simulink model "Battery_50kw_AC_500KW_400V_pruebas_2020_2_individual"  (R2020b)
settings: Solver=VariableStepAuto  StartTime=0.0  StopTime=0.4  RelTol=1e-3
InitFcn:
  | Ts=100e-6;
  | Timer=0.001;
StartFcn:
  | Ts=100e-6;
  | Timer=0.001;
undefined symbols (not defined in the file or in its folder): Ion, Lithium
libraries: powerlib x44, powerlib_meascontrol x16, slpidlib x10, simulink x5, electricdrivelib x1
(part 2 of 2)

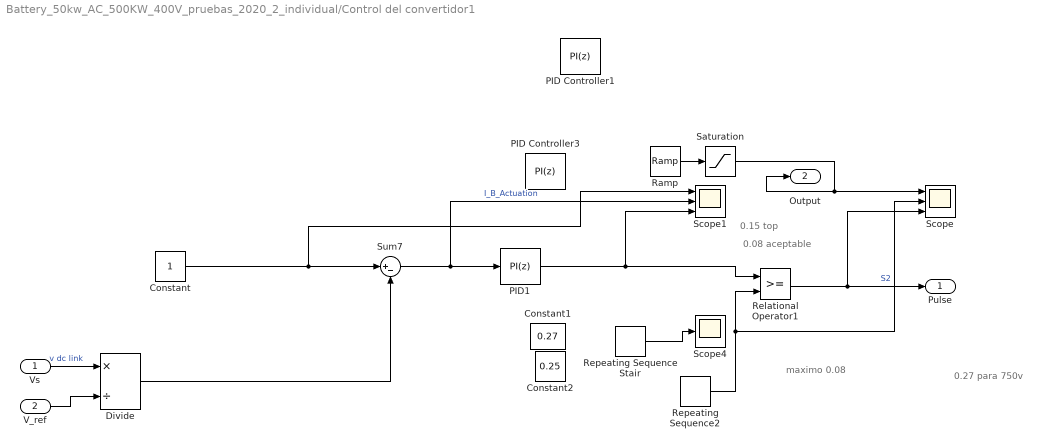
== system Battery_50kw_AC_500KW_400V_pruebas_2020_2_individual/Control del convertidor1 ==
  note: 0.08 aceptable
  note: 0.15 top
  note: 0.27 para 750v
  note: maximo 0.08
  Vs : Inport
  V_ref : Inport  Port=2
  Constant : Constant
  Constant1 : Constant  Value=0.27
  Constant2 : Constant  Value=0.25
  Divide : Product  Inputs=*/
  PID Controller1 : slpidlib/PID Controller  Controller=PI  Form=Parallel  TimeDomain=Discrete-time  UseExternalTs=off  SampleTime=Ts  IntegratorMethod=Forward Euler  FilterMethod=Forward Euler  ControllerParametersSource=internal  P=0.01  I=0.02  D=0  UseFilter=on  N=100  TunerSelectOption=Transfer Function Based (PID Tuner App)  InitialConditionSource=internal  InitialConditionForIntegrator=0  InitialConditionForFilter=0  DifferentiatorICPrevScaledInput=0  ExternalReset=none  TrackingMode=off  Kt=1  LimitOutput=on  SatLimitsSource=internal  UpperSaturationLimit=0.95  LowerSaturationLimit=0  LinearizeAsGain=on  AntiWindupMode=clamping  Kb=1  POutMin=[]  POutMax=[]  IOutMin=[]  IOutMax=[]  DOutMin=[]  DOutMax=[]  NOutMin=[]  NOutMax=[]  SumOutMin=[]  SumOutMax=[]  SaturationOutMin=[]  SaturationOutMax=[]  PParamMin=[]  PParamMax=[]  IParamMin=[]  IParamMax=[]  DParamMin=[]  DParamMax=[]  NParamMin=[]  NParamMax=[]  KbParamMin=[]  KbParamMax=[]  KtParamMin=[]  KtParamMax=[]  KbOutMin=[]  KbOutMax=[]  KtOutMin=[]  KtOutMax=[]  IntegratorOutMin=[]  IntegratorOutMax=[]  FilterOutMin=[]  FilterOutMax=[]  SumI1OutMin=[]  SumI1OutMax=[]  SumI2OutMin=[]  SumI2OutMax=[]  SumI3OutMin=[]  SumI3OutMax=[]  SumI4OutMin=[]  SumI4OutMax=[]  SumDOutMin=[]  SumDOutMax=[]  DifferentiatorOutMin=[]  DifferentiatorOutMax=[]  FilterDiffOutCoefMin=[]  FilterDiffOutCoefMax=[]  ReciprocalOutMin=[]  ReciprocalOutMax=[]  SumDenOutMin=[]  SumDenOutMax=[]  SumNumOutMin=[]  SumNumOutMax=[]  DivideOutMin=[]  DivideOutMax=[]  UdiffTsProdOutMin=[]  UdiffTsProdOutMax=[]  NTsProdOutMin=[]  NTsProdOutMax=[]  UintegralTsProdOutMin=[]  UintegralTsProdOutMax=[]  UngainTsProdOutMin=[]  UngainTsProdOutMax=[]  IntegratorContinuousStateAttributes=''  IntegratorStateMustResolveToSignalObject=off  IntegratorRTWStateStorageClass=Auto  FilterContinuousStateAttributes=''  FilterStateMustResolveToSignalObject=off  FilterRTWStateStorageClass=Auto  ParallelPVariant=InternalParameters  IdealPVariant=Disabled  IVariant=InternalParameters  DVariant=Disabled  IntegratorVariant=Discrete  SatVariant=Enabled  AWVariant=DiscClampingParallel  PCopyVariant=Disabled  TRVariant=Disabled  FdbkBlocksVariant=Forward  IdealPFdbkVariant=Disabled  SatFdbkVariant=Disabled  DerivativeFilterVariant=Disabled  NVariant=Disabled  NCopyVariant=Disabled_SignalSpec  FilterICVariant=Disabled  IntegratorICVariant=InternalICs  ExternalResetVariant=Disabled  TRSumVariant=Passthrough  SumFdbkVariant=Disabled  SumVariant=Sum_PI  TsampFilterVariant=InternalTs  TsampNgainVariant=Passthrough  TsampIntegralVariant=Passthrough  ExternalSaturationOutDataTypeStr=Inherit: Same as second input
  PID Controller3 : slpidlib/PID Controller  Controller=PI  Form=Parallel  TimeDomain=Discrete-time  UseExternalTs=off  SampleTime=Ts  IntegratorMethod=Forward Euler  FilterMethod=Forward Euler  ControllerParametersSource=internal  P=0.001  I=0.02  D=0  UseFilter=on  N=100  TunerSelectOption=Transfer Function Based (PID Tuner App)  InitialConditionSource=internal  InitialConditionForIntegrator=0  InitialConditionForFilter=0  DifferentiatorICPrevScaledInput=0  ExternalReset=none  TrackingMode=off  Kt=1  LimitOutput=on  SatLimitsSource=internal  UpperSaturationLimit=0.95  LowerSaturationLimit=0  LinearizeAsGain=on  AntiWindupMode=clamping  Kb=1  POutMin=[]  POutMax=[]  IOutMin=[]  IOutMax=[]  DOutMin=[]  DOutMax=[]  NOutMin=[]  NOutMax=[]  SumOutMin=[]  SumOutMax=[]  SaturationOutMin=[]  SaturationOutMax=[]  PParamMin=[]  PParamMax=[]  IParamMin=[]  IParamMax=[]  DParamMin=[]  DParamMax=[]  NParamMin=[]  NParamMax=[]  KbParamMin=[]  KbParamMax=[]  KtParamMin=[]  KtParamMax=[]  KbOutMin=[]  KbOutMax=[]  KtOutMin=[]  KtOutMax=[]  IntegratorOutMin=[]  IntegratorOutMax=[]  FilterOutMin=[]  FilterOutMax=[]  SumI1OutMin=[]  SumI1OutMax=[]  SumI2OutMin=[]  SumI2OutMax=[]  SumI3OutMin=[]  SumI3OutMax=[]  SumI4OutMin=[]  SumI4OutMax=[]  SumDOutMin=[]  SumDOutMax=[]  DifferentiatorOutMin=[]  DifferentiatorOutMax=[]  FilterDiffOutCoefMin=[]  FilterDiffOutCoefMax=[]  ReciprocalOutMin=[]  ReciprocalOutMax=[]  SumDenOutMin=[]  SumDenOutMax=[]  SumNumOutMin=[]  SumNumOutMax=[]  DivideOutMin=[]  DivideOutMax=[]  UdiffTsProdOutMin=[]  UdiffTsProdOutMax=[]  NTsProdOutMin=[]  NTsProdOutMax=[]  UintegralTsProdOutMin=[]  UintegralTsProdOutMax=[]  UngainTsProdOutMin=[]  UngainTsProdOutMax=[]  IntegratorContinuousStateAttributes=''  IntegratorStateMustResolveToSignalObject=off  IntegratorRTWStateStorageClass=Auto  FilterContinuousStateAttributes=''  FilterStateMustResolveToSignalObject=off  FilterRTWStateStorageClass=Auto  ParallelPVariant=InternalParameters  IdealPVariant=Disabled  IVariant=InternalParameters  DVariant=Disabled  IntegratorVariant=Discrete  SatVariant=Enabled  AWVariant=DiscClampingParallel  PCopyVariant=Disabled  TRVariant=Disabled  FdbkBlocksVariant=Forward  IdealPFdbkVariant=Disabled  SatFdbkVariant=Disabled  DerivativeFilterVariant=Disabled  NVariant=Disabled  NCopyVariant=Disabled_SignalSpec  FilterICVariant=Disabled  IntegratorICVariant=InternalICs  ExternalResetVariant=Disabled  TRSumVariant=Passthrough  SumFdbkVariant=Disabled  SumVariant=Sum_PI  TsampFilterVariant=InternalTs  TsampNgainVariant=Passthrough  TsampIntegralVariant=Passthrough  ExternalSaturationOutDataTypeStr=Inherit: Same as second input
  PID1 : slpidlib/PID Controller  Controller=PI  Form=Parallel  TimeDomain=Discrete-time  UseExternalTs=off  SampleTime=Ts  IntegratorMethod=Forward Euler  FilterMethod=Forward Euler  ControllerParametersSource=internal  P=0.7  I=5  D=0  UseFilter=on  N=100  TunerSelectOption=Transfer Function Based (PID Tuner App)  InitialConditionSource=internal  InitialConditionForIntegrator=0.26  InitialConditionForFilter=0  DifferentiatorICPrevScaledInput=0  ExternalReset=none  TrackingMode=off  Kt=1  LimitOutput=on  SatLimitsSource=internal  UpperSaturationLimit=0.97  LowerSaturationLimit=0  LinearizeAsGain=on  AntiWindupMode=clamping  Kb=1  POutMin=[]  POutMax=[]  IOutMin=[]  IOutMax=[]  DOutMin=[]  DOutMax=[]  NOutMin=[]  NOutMax=[]  SumOutMin=[]  SumOutMax=[]  SaturationOutMin=[]  SaturationOutMax=[]  PParamMin=[]  PParamMax=[]  IParamMin=[]  IParamMax=[]  DParamMin=[]  DParamMax=[]  NParamMin=[]  NParamMax=[]  KbParamMin=[]  KbParamMax=[]  KtParamMin=[]  KtParamMax=[]  KbOutMin=[]  KbOutMax=[]  KtOutMin=[]  KtOutMax=[]  IntegratorOutMin=[]  IntegratorOutMax=[]  FilterOutMin=[]  FilterOutMax=[]  SumI1OutMin=[]  SumI1OutMax=[]  SumI2OutMin=[]  SumI2OutMax=[]  SumI3OutMin=[]  SumI3OutMax=[]  SumI4OutMin=[]  SumI4OutMax=[]  SumDOutMin=[]  SumDOutMax=[]  DifferentiatorOutMin=[]  DifferentiatorOutMax=[]  FilterDiffOutCoefMin=[]  FilterDiffOutCoefMax=[]  ReciprocalOutMin=[]  ReciprocalOutMax=[]  SumDenOutMin=[]  SumDenOutMax=[]  SumNumOutMin=[]  SumNumOutMax=[]  DivideOutMin=[]  DivideOutMax=[]  UdiffTsProdOutMin=[]  UdiffTsProdOutMax=[]  NTsProdOutMin=[]  NTsProdOutMax=[]  UintegralTsProdOutMin=[]  UintegralTsProdOutMax=[]  UngainTsProdOutMin=[]  UngainTsProdOutMax=[]  IntegratorContinuousStateAttributes=''  IntegratorStateMustResolveToSignalObject=off  IntegratorRTWStateStorageClass=Auto  FilterContinuousStateAttributes=''  FilterStateMustResolveToSignalObject=off  FilterRTWStateStorageClass=Auto  ParallelPVariant=InternalParameters  IdealPVariant=Disabled  IVariant=InternalParameters  DVariant=Disabled  IntegratorVariant=Discrete  SatVariant=Enabled  AWVariant=DiscClampingParallel  PCopyVariant=Disabled  TRVariant=Disabled  FdbkBlocksVariant=Forward  IdealPFdbkVariant=Disabled  SatFdbkVariant=Disabled  DerivativeFilterVariant=Disabled  NVariant=Disabled  NCopyVariant=Disabled_SignalSpec  FilterICVariant=Disabled  IntegratorICVariant=InternalICs  ExternalResetVariant=Disabled  TRSumVariant=Passthrough  SumFdbkVariant=Disabled  SumVariant=Sum_PI  TsampFilterVariant=InternalTs  TsampNgainVariant=Passthrough  TsampIntegralVariant=Passthrough  ExternalSaturationOutDataTypeStr=Inherit: Same as second input
  Ramp : simulink/Sources/Ramp  slope=0.9  start=0  InitialOutput=0.6
  Relational Operator1 : RelationalOperator  OutDataTypeStr=boolean  RndMeth=Nearest
  Repeating Sequence Stair : simulink/Sources/Repeating Sequence Stair  OutValues=[0.2 0.21 0.22 0.23 0.24 0.25].'  tsamp=0.05  OutMin=[]  OutMax=[]  OutDataTypeStr=double  OutputDataTypeScalingMode=double  OutDataType=fixdt(0,8)  ConRadixGroup=Best Precision: Vector-wise  OutScaling=2^-12
  Repeating Sequence2 : simulink/Sources/Repeating Sequence  rep_seq_t=[0 Ts/2 Ts]  rep_seq_y=[0 1 0]
  Saturation : Saturate  UpperLimit=1  LowerLimit=0
  Scope : Scope  NumInputPorts=3
  Scope1 : Scope  NumInputPorts=3
  Scope4 : Scope
  Sum7 : Sum  Inputs=|+-
  Pulse : Outport
  Output : Outport  Port=2
  wires:
  Sum7/1 -> Scope1/2, PID1/1  "I_B_Actuation"
  Relational Operator1/1 -> Pulse/1, Scope/3  "S2"
  Ramp/1 -> Saturation/1
  Repeating Sequence2/1 -> Scope/2, Relational Operator1/2
  Constant/1 -> Scope1/1, Sum7/1
  Vs/1 -> Divide/1  "v dc link"
  V_ref/1 -> Divide/2
  Divide/1 -> Sum7/2
  Saturation/1 -> Output/1, Scope/1
  Repeating Sequence Stair/1 -> Scope4/1
  PID1/1 -> Scope1/3, Relational Operator1/1

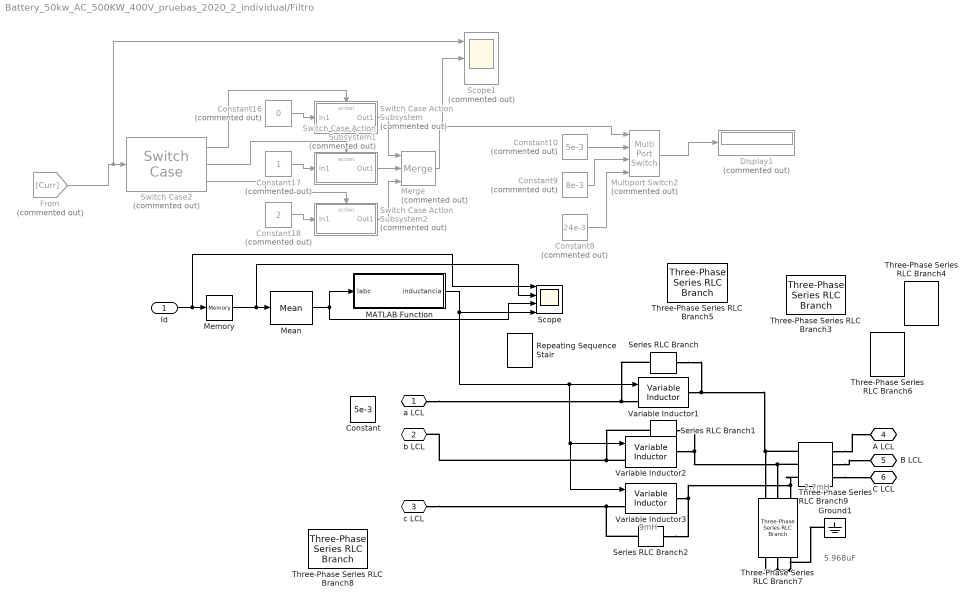
== system Battery_50kw_AC_500KW_400V_pruebas_2020_2_individual/Filtro ==
  note: 2.7mH
  note: 9mH
  note: 5.968uF
  Id : Inport
  Constant : Constant  Value=5e-3
  Constant10 : Constant  Commented=on  Value=5e-3
  Constant16 : Constant  Commented=on  Value=0
  Constant17 : Constant  Commented=on
  Constant18 : Constant  Commented=on  Value=2
  Constant8 : Constant  Commented=on  Value=24e-3
  Constant9 : Constant  Commented=on  Value=8e-3
  Display1 : Display  Commented=on
  From : From  Commented=on  GotoTag=Curr
  Ground1 : powerlib/Elements/Ground  LConnTagsString=a
  MATLAB Function : MATLAB Function  TreatAsAtomicUnit=on
  Mean : powerlib_meascontrol/Measurements/Mean  Freq=60  Vinit=0  Ts=0
  Memory : Memory
  Merge : Merge  Commented=on  Inputs=3
  Multiport Switch2 : MultiPortSwitch  Commented=on  DataPortOrder=Zero-based contiguous  zeroidx=on  InputSameDT=on
  Repeating Sequence Stair : simulink/Sources/Repeating Sequence Stair  OutValues=[24e-3 8e-3 5e-3 8e-3 ].'  tsamp=0.05  OutMin=[]  OutMax=[]  OutDataTypeStr=double  OutputDataTypeScalingMode=double  OutDataType=fixdt(0,8)  ConRadixGroup=Best Precision: Vector-wise  OutScaling=2^-12
  Scope : Scope  NumInputPorts=4
  Scope1 : Scope  Commented=on  NumInputPorts=3
  Series RLC Branch : powerlib/Elements/Series RLC Branch  LConnTagsString=__new0  RConnTagsString=__new0  BranchType=R  Resistance=70  Inductance=1e-3  SetiL0=off  InitialCurrent=0  Capacitance=1e-6  Setx0=off  InitialVoltage=0  Measurements=None
  Series RLC Branch1 : powerlib/Elements/Series RLC Branch  LConnTagsString=__new0  RConnTagsString=__new0  BranchType=R  Resistance=70  Inductance=1e-3  SetiL0=off  InitialCurrent=0  Capacitance=1e-6  Setx0=off  InitialVoltage=0  Measurements=None
  Series RLC Branch2 : powerlib/Elements/Series RLC Branch  LConnTagsString=__new0  RConnTagsString=__new0  BranchType=R  Resistance=70  Inductance=1e-3  SetiL0=off  InitialCurrent=0  Capacitance=1e-6  Setx0=off  InitialVoltage=0  Measurements=None
  Switch Case Action Subsystem : Subsystem  Commented=on  TreatAsAtomicUnit=on
  Switch Case Action Subsystem1 : Subsystem  Commented=on  TreatAsAtomicUnit=on
  Switch Case Action Subsystem2 : Subsystem  Commented=on  TreatAsAtomicUnit=on
  Switch Case2 : SwitchCase  Commented=on  CaseConditions={[75:100],[45:70]}
  Three-Phase Series RLC Branch3 : powerlib/Elements/Three-Phase Series RLC Branch  LConnTagsString=A|B|C  RConnTagsString=A|B|C  BranchType=L  Resistance=1  Inductance=3.186e-3  Capacitance=1e-6  Measurements=None
  Three-Phase Series RLC Branch4 : powerlib/Elements/Three-Phase Series RLC Branch  LConnTagsString=A|B|C  RConnTagsString=A|B|C  BranchType=L  Resistance=1  Inductance=1.186e-3  Capacitance=1e-6  Measurements=None
  Three-Phase Series RLC Branch5 : powerlib/Elements/Three-Phase Series RLC Branch  LConnTagsString=A|B|C  RConnTagsString=A|B|C  BranchType=L  Resistance=1  Inductance=4.186e-3  Capacitance=1e-6  Measurements=None
  Three-Phase Series RLC Branch6 : powerlib/Elements/Three-Phase Series RLC Branch  LConnTagsString=A|B|C  RConnTagsString=A|B|C  BranchType=L  Resistance=1  Inductance=1.186e-3  Capacitance=1e-6  Measurements=None
  Three-Phase Series RLC Branch7 : powerlib/Elements/Three-Phase Series RLC Branch  LConnTagsString=A|B|C  RConnTagsString=A|B|C  BranchType=C  Resistance=1  Inductance=1e-3  Capacitance=1.8236e-5  Measurements=None
  Three-Phase Series RLC Branch8 : powerlib/Elements/Three-Phase Series RLC Branch  LConnTagsString=A|B|C  RConnTagsString=A|B|C  BranchType=L  Resistance=1  Inductance=5.586e-3  Capacitance=1e-6  Measurements=None
  Three-Phase Series RLC Branch9 : powerlib/Elements/Three-Phase Series RLC Branch  LConnTagsString=A|B|C  RConnTagsString=A|B|C  BranchType=L  Resistance=1  Inductance=0.100e-3  Capacitance=1e-6  Measurements=None
  Variable Inductor1 : powerlib/Elements/Variable Inductor  methode=Backward Euler  Labsmin=1e-6  Initialize=off  iL0=1  L0=24e-3  Vl0=2.2768e-16
      settings: SourceProductBaseCode=PS
  Variable Inductor2 : powerlib/Elements/Variable Inductor  methode=Backward Euler  Labsmin=1e-6  Initialize=off  iL0=1  L0=24e-3  Vl0=-3.2526e-17
      settings: SourceProductBaseCode=PS
  Variable Inductor3 : powerlib/Elements/Variable Inductor  methode=Backward Euler  Labsmin=1e-6  Initialize=off  iL0=1  L0=24e-3  Vl0=-3.2526e-17
      settings: SourceProductBaseCode=PS
  a LCL : PMIOPort  Side=Right
  "b LCL " : PMIOPort  Port=2  Side=Right
  c LCL : PMIOPort  Port=3  Side=Right
  A LCL : PMIOPort  Port=4  Side=Left
  B LCL : PMIOPort  Port=5  Side=Left
  C LCL : PMIOPort  Port=6  Side=Left
  wires:
  Constant17/1 -> Switch Case Action Subsystem1/1(In1)
  Constant18/1 -> Switch Case Action Subsystem2/1(In1)
  From/1 -> Scope1/1, Switch Case2/1
  Switch Case2/3 -> Switch Case Action Subsystem2/Action
  Switch Case2/2 -> Switch Case Action Subsystem1/Action
  Constant16/1 -> Switch Case Action Subsystem/1(In1)
  Switch Case2/1 -> Switch Case Action Subsystem/Action
  Constant10/1 -> Multiport Switch2/2
  Constant9/1 -> Multiport Switch2/3
  Constant8/1 -> Multiport Switch2/4
  Switch Case Action Subsystem/1(Out1) -> Merge/1
  Switch Case Action Subsystem1/1(Out1) -> Merge/2
  Switch Case Action Subsystem2/1(Out1) -> Merge/3
  Merge/1 -> Scope1/2, Multiport Switch2/1
  Multiport Switch2/1 -> Display1/1
  Id/1 -> Scope/1, Memory/1
  MATLAB Function/1(inductancia) -> Scope/4, Variable Inductor3/1, Variable Inductor2/1, Variable Inductor1/1
  Memory/1 -> Scope/2, Mean/1
  Mean/1 -> MATLAB Function/1(Iabc), Scope/3
  connections:
  Three-Phase Series RLC Branch9/LConn3 -- C LCL/RConn1
  Three-Phase Series RLC Branch9/LConn1 -- A LCL/RConn1
  Three-Phase Series RLC Branch9/LConn2 -- B LCL/RConn1
  Variable Inductor2/LConn1 -- Series RLC Branch1/LConn1 -- "b LCL "/RConn1
  a LCL/RConn1 -- Series RLC Branch/LConn1 -- Variable Inductor1/LConn1
  Three-Phase Series RLC Branch9/RConn3 -- Series RLC Branch2/RConn1 -- Variable Inductor3/RConn1 -- Three-Phase Series RLC Branch7/LConn3
  c LCL/RConn1 -- Series RLC Branch2/LConn1 -- Variable Inductor3/LConn1
  Three-Phase Series RLC Branch9/RConn2 -- Series RLC Branch1/RConn1 -- Variable Inductor2/RConn1 -- Three-Phase Series RLC Branch7/LConn2
  Three-Phase Series RLC Branch9/RConn1 -- Series RLC Branch/RConn1 -- Variable Inductor1/RConn1 -- Three-Phase Series RLC Branch7/LConn1
  Three-Phase Series RLC Branch7/RConn2 -- Three-Phase Series RLC Branch7/RConn3 -- Ground1/LConn1 -- Three-Phase Series RLC Branch7/RConn1

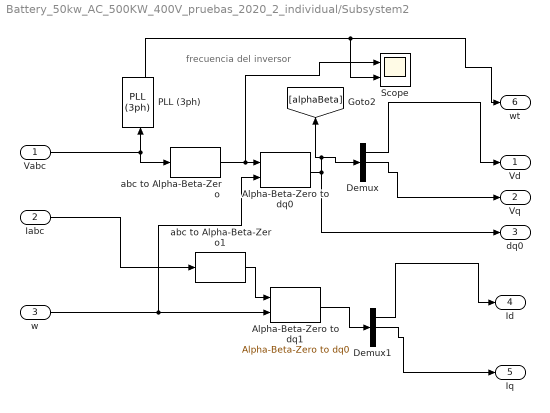
== system Battery_50kw_AC_500KW_400V_pruebas_2020_2_individual/Subsystem2 ==
  note: frecuencia del inversor
  Vabc : Inport
  Iabc : Inport  Port=2
  w : Inport  Port=3
  Alpha-Beta-Zero to dq0 : powerlib_meascontrol/Transformations/Alpha-Beta-Zero to dq0  Alignment=90 degrees behind phase A axis
  Alpha-Beta-Zero to dq1 : powerlib_meascontrol/Transformations/Alpha-Beta-Zero to dq0  Alignment=90 degrees behind phase A axis
  Demux : Demux  Outputs=3
  Demux1 : Demux  Outputs=3
  PLL (3ph) : powerlib_meascontrol/PLL/PLL (3ph)  Fmin=45  Par_Init=[0, 50]  ParK=[180, 3200, 1]  TcD=1e-4  MaxRateChangeFreq=12  FilterCutOffFreq=25  Ts=0  AGC=on
  Scope : Scope  NumInputPorts=2
  abc to Alpha-Beta-Zero : powerlib_meascontrol/Transformations/abc to Alpha-Beta-Zero
  abc to Alpha-Beta-Zero1 : powerlib_meascontrol/Transformations/abc to Alpha-Beta-Zero
  Vd : Outport
  Vq : Outport  Port=2
  dq0 : Outport  Port=3
  Id : Outport  Port=4
  Iq : Outport  Port=5
  wt : Outport  Port=6
  wires:
  Demux/2 -> Vq/1
  Demux1/1 -> Id/1
  Demux1/2 -> Iq/1
  Alpha-Beta-Zero to dq0/1 -> dq0/1, Demux/1, [alphaBeta]
  abc to Alpha-Beta-Zero/1 -> Scope/1, Alpha-Beta-Zero to dq0/1
  abc to Alpha-Beta-Zero1/1 -> Alpha-Beta-Zero to dq1/1
  Alpha-Beta-Zero to dq1/1 -> Demux1/1
  Vabc/1 -> PLL (3ph)/1, abc to Alpha-Beta-Zero/1
  w/1 -> Alpha-Beta-Zero to dq0/2, Alpha-Beta-Zero to dq1/2
  Demux/1 -> Vd/1
  Iabc/1 -> abc to Alpha-Beta-Zero1/1
  PLL (3ph)/2 -> wt/1, Scope/2

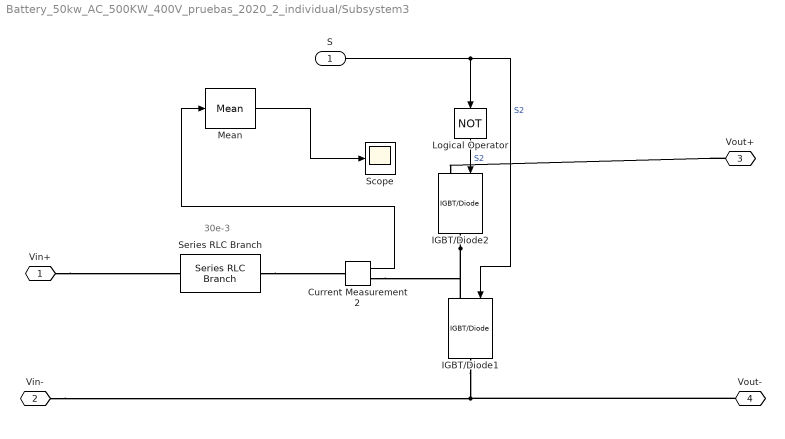
== system Battery_50kw_AC_500KW_400V_pruebas_2020_2_individual/Subsystem3 ==
  note: 30e-3
  S : Inport
  Current Measurement2 : powerlib/Measurements/Current Measurement  PhasorSimulation=off  OutputType=Complex  PSBequivalent=0
  IGBT/Diode1 : powerlib/Power Electronics/IGBT//Diode  Ron=1e-3  Rs=1e5  Cs=inf  Measurements=off
  IGBT/Diode2 : powerlib/Power Electronics/IGBT//Diode  Ron=1e-3  Rs=1e5  Cs=inf  Measurements=off
  Logical Operator : Logic  Operator=NOT  AllPortsSameDT=off  OutDataTypeStr=boolean
  Mean : powerlib_meascontrol/Measurements/Mean  Freq=60  Vinit=0  Ts=0
  Scope : Scope
  Series RLC Branch : powerlib/Elements/Series RLC Branch  LConnTagsString=__new0  RConnTagsString=__new0  BranchType=L  Resistance=3  Inductance=3.1e-6  SetiL0=off  InitialCurrent=0  Capacitance=1e-6  Setx0=off  InitialVoltage=0  Measurements=None
  Vin+ : PMIOPort  Side=Left
  Vin- : PMIOPort  Port=2  Side=Left
  Vout+ : PMIOPort  Port=3  Side=Right
  Vout- : PMIOPort  Port=4  Side=Right
  wires:
  Current Measurement2/1 -> Mean/1
  Logical Operator/1 -> IGBT/Diode2/1  "S2"
  S/1 -> Logical Operator/1, IGBT/Diode1/1  "S2"
  Mean/1 -> Scope/1
  connections:
  Vout+/RConn1 -- IGBT/Diode2/LConn1
  IGBT/Diode2/RConn1 -- Current Measurement2/RConn1 -- IGBT/Diode1/LConn1
  Vin+/RConn1 -- Series RLC Branch/LConn1
  Series RLC Branch/RConn1 -- Current Measurement2/LConn1
  IGBT/Diode1/RConn1 -- Vout-/RConn1 -- Vin-/RConn1

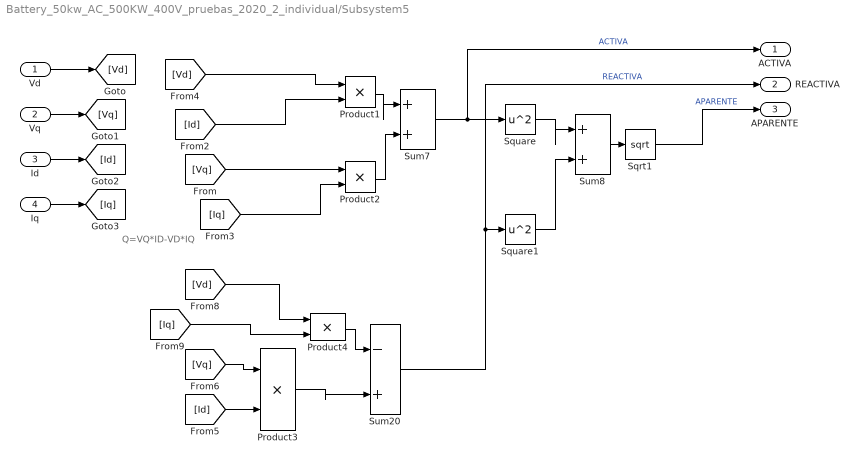
== system Battery_50kw_AC_500KW_400V_pruebas_2020_2_individual/Subsystem5 ==
  note: Q=VQ*ID-VD*IQ
  Vd : Inport
  Vq : Inport  Port=2
  Id : Inport  Port=3
  Iq : Inport  Port=4
  Product{1..4} (4 alike) : Product
  Sqrt1 : Sqrt  SaturateOnIntegerOverflow=on
  Square : Math  Operator=square  SaturateOnIntegerOverflow=on
  Square1 : Math  Operator=square  SaturateOnIntegerOverflow=on
  Sum20 : Sum  Inputs=|-+
  Sum7 : Sum  Inputs=|++
  Sum8 : Sum  Inputs=|++
  ACTIVA : Outport
  REACTIVA : Outport  Port=2
  APARENTE : Outport  Port=3
  wires:
  Product1/1 -> Sum7/1
  Product2/1 -> Sum7/2
  Square/1 -> Sum8/1
  Sum7/1 -> ACTIVA/1, Square/1  "ACTIVA"
  Sum8/1 -> Sqrt1/1
  [Iq] -> Product2/2
  [Vq] -> Product2/1
  [Vd] -> Product1/1
  Sqrt1/1 -> APARENTE/1  "APARENTE"
  Sum20/1 -> REACTIVA/1, Square1/1  "REACTIVA"
  Square1/1 -> Sum8/2
  Product4/1 -> Sum20/1
  [Vd] -> Product4/1
  [Vq] -> Product3/1
  Product3/1 -> Sum20/2
  [Id] -> Product3/2
  [Id] -> Product1/2
  Iq/1 -> [Iq]
  Id/1 -> [Id]
  Vq/1 -> [Vq]
  Vd/1 -> [Vd]
  [Iq] -> Product4/2

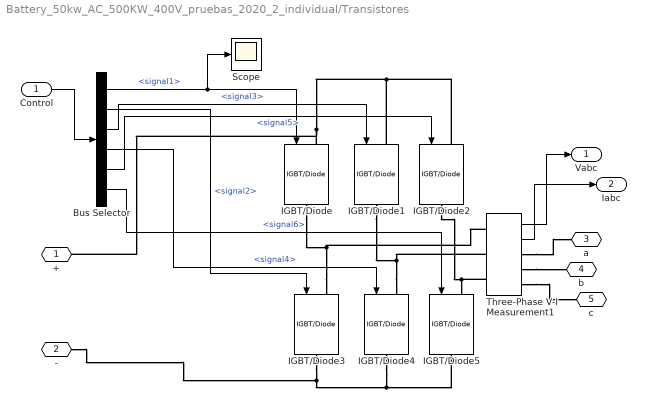
== system Battery_50kw_AC_500KW_400V_pruebas_2020_2_individual/Transistores ==
  Control : Inport
  Bus Selector : BusSelector  OutputSignals=signal1,signal2,signal3,signal4,signal5,signal6
  IGBT/Diode{,1..5} (6 alike) : powerlib/Power Electronics/IGBT//Diode  Ron=1e-3  Rs=1e5  Cs=inf  Measurements=off
  Scope : Scope
  Three-Phase V-I Measurement1 : powerlib/Measurements/Three-Phase V-I Measurement  VoltageMeasurement=phase-to-phase  SetLabelV=off  LabelV=Vabc  Vpu=off  VpuLL=off  CurrentMeasurement=yes  SetLabelI=off  LabelI=Iabc  Ipu=off  Pbase=100e6  Vbase=500e3  OutputType=Complex  PhasorSimulation=off  PSBequivalent=0
  + : PMIOPort  Side=Left
  - : PMIOPort  Port=2  Side=Left
  a : PMIOPort  Port=3  Side=Right
  b : PMIOPort  Port=4  Side=Right
  c : PMIOPort  Port=5  Side=Right
  Vabc : Outport
  Iabc : Outport  Port=2
  wires:
  Bus Selector/6 -> IGBT/Diode5/1  "<signal6>"
  Bus Selector/5 -> IGBT/Diode2/1  "<signal5>"
  Bus Selector/4 -> IGBT/Diode4/1  "<signal4>"
  Bus Selector/3 -> IGBT/Diode1/1  "<signal3>"
  Bus Selector/2 -> IGBT/Diode3/1  "<signal2>"
  Control/1 -> Bus Selector/1
  Bus Selector/1 -> Scope/1, IGBT/Diode/1  "<signal1>"
  Three-Phase V-I Measurement1/1 -> Vabc/1
  Three-Phase V-I Measurement1/2 -> Iabc/1
  connections:
  Three-Phase V-I Measurement1/RConn2 -- b/RConn1
  Three-Phase V-I Measurement1/RConn1 -- a/RConn1
  Three-Phase V-I Measurement1/RConn3 -- c/RConn1
  IGBT/Diode5/RConn1 -- IGBT/Diode4/RConn1 -- -/RConn1 -- IGBT/Diode3/RConn1
  +/RConn1 -- IGBT/Diode/LConn1 -- IGBT/Diode2/LConn1 -- IGBT/Diode1/LConn1
  IGBT/Diode5/LConn1 -- Three-Phase V-I Measurement1/LConn3 -- IGBT/Diode2/RConn1
  IGBT/Diode4/LConn1 -- Three-Phase V-I Measurement1/LConn2 -- IGBT/Diode1/RConn1
  IGBT/Diode3/LConn1 -- Three-Phase V-I Measurement1/LConn1 -- IGBT/Diode/RConn1

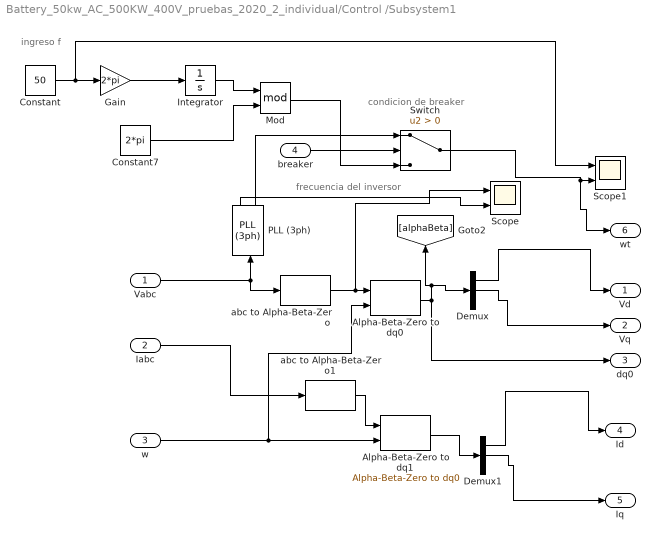
== system Battery_50kw_AC_500KW_400V_pruebas_2020_2_individual/Control /Subsystem1 ==
  note: frecuencia del inversor
  note: condicion de breaker
  note: ingreso f
  Vabc : Inport
  Iabc : Inport  Port=2
  w : Inport  Port=3
  breaker : Inport  Port=4
  Alpha-Beta-Zero to dq0 : powerlib_meascontrol/Transformations/Alpha-Beta-Zero to dq0  Alignment=90 degrees behind phase A axis
  Alpha-Beta-Zero to dq1 : powerlib_meascontrol/Transformations/Alpha-Beta-Zero to dq0  Alignment=90 degrees behind phase A axis
  Constant : Constant  Value=50
  Constant7 : Constant  Value=2*pi
  Demux : Demux  Outputs=3
  Demux1 : Demux  Outputs=3
  Gain : Gain  Gain=2*pi
  Integrator : Integrator
  Mod : Math  Operator=mod  SaturateOnIntegerOverflow=on
  PLL (3ph) : powerlib_meascontrol/PLL/PLL (3ph)  Fmin=45  Par_Init=[0, 50]  ParK=[180, 3200, 1]  TcD=1e-4  MaxRateChangeFreq=12  FilterCutOffFreq=25  Ts=0  AGC=on
  Scope : Scope  NumInputPorts=2
  Scope1 : Scope  NumInputPorts=2
  Switch : Switch  Criteria=u2 > Threshold
  abc to Alpha-Beta-Zero : powerlib_meascontrol/Transformations/abc to Alpha-Beta-Zero
  abc to Alpha-Beta-Zero1 : powerlib_meascontrol/Transformations/abc to Alpha-Beta-Zero
  Vd : Outport
  Vq : Outport  Port=2
  dq0 : Outport  Port=3
  Id : Outport  Port=4
  Iq : Outport  Port=5
  wt : Outport  Port=6
  wires:
  Iabc/1 -> abc to Alpha-Beta-Zero1/1
  Demux/1 -> Vd/1
  w/1 -> Alpha-Beta-Zero to dq1/2, Alpha-Beta-Zero to dq0/2
  Vabc/1 -> abc to Alpha-Beta-Zero/1, PLL (3ph)/1
  Alpha-Beta-Zero to dq1/1 -> Demux1/1
  abc to Alpha-Beta-Zero1/1 -> Alpha-Beta-Zero to dq1/1
  abc to Alpha-Beta-Zero/1 -> Alpha-Beta-Zero to dq0/1, Scope/1
  Alpha-Beta-Zero to dq0/1 -> [alphaBeta], Demux/1, dq0/1
  Demux1/2 -> Iq/1
  Demux1/1 -> Id/1
  Demux/2 -> Vq/1
  Switch/1 -> wt/1, Scope1/2
  Constant/1 -> Gain/1, Scope1/1
  Gain/1 -> Integrator/1
  breaker/1 -> Switch/2
  PLL (3ph)/2 -> Switch/1
  Constant7/1 -> Mod/2
  Integrator/1 -> Mod/1
  Mod/1 -> Switch/3
  PLL (3ph)/1 -> Scope/2

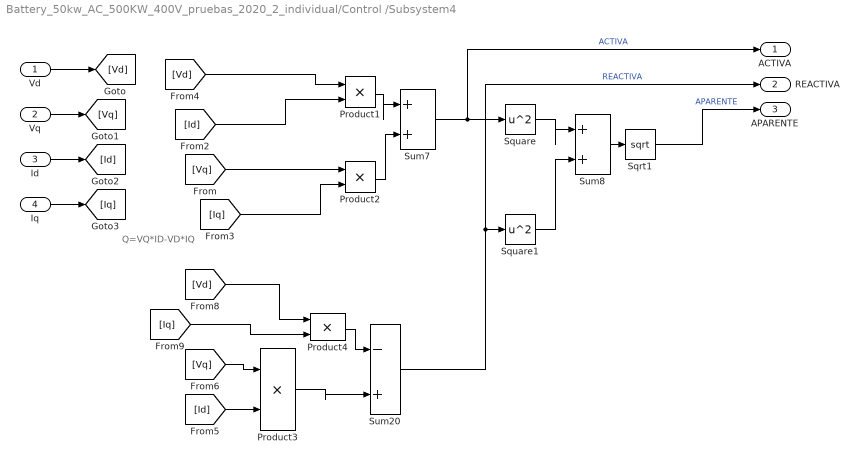
== system Battery_50kw_AC_500KW_400V_pruebas_2020_2_individual/Control /Subsystem4 ==
  note: Q=VQ*ID-VD*IQ
  Vd : Inport
  Vq : Inport  Port=2
  Id : Inport  Port=3
  Iq : Inport  Port=4
  Product{1..4} (4 alike) : Product
  Sqrt1 : Sqrt  SaturateOnIntegerOverflow=on
  Square : Math  Operator=square  SaturateOnIntegerOverflow=on
  Square1 : Math  Operator=square  SaturateOnIntegerOverflow=on
  Sum20 : Sum  Inputs=|-+
  Sum7 : Sum  Inputs=|++
  Sum8 : Sum  Inputs=|++
  ACTIVA : Outport
  REACTIVA : Outport  Port=2
  APARENTE : Outport  Port=3
  wires:
  [Iq] -> Product4/2
  Vd/1 -> [Vd]
  Vq/1 -> [Vq]
  Id/1 -> [Id]
  Iq/1 -> [Iq]
  [Id] -> Product1/2
  [Id] -> Product3/2
  Product3/1 -> Sum20/2
  [Vq] -> Product3/1
  [Vd] -> Product4/1
  Product4/1 -> Sum20/1
  Square1/1 -> Sum8/2
  Sum20/1 -> Square1/1, REACTIVA/1  "REACTIVA"
  Sqrt1/1 -> APARENTE/1  "APARENTE"
  [Vd] -> Product1/1
  [Vq] -> Product2/1
  [Iq] -> Product2/2
  Sum8/1 -> Sqrt1/1
  Sum7/1 -> Square/1, ACTIVA/1  "ACTIVA"
  Square/1 -> Sum8/1
  Product2/1 -> Sum7/2
  Product1/1 -> Sum7/1

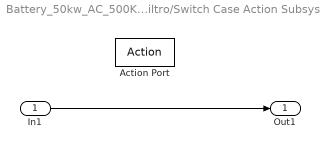
== system Battery_50kw_AC_500KW_400V_pruebas_2020_2_individual/Filtro/Switch Case Action Subsystem ==
  In1 : Inport
  Action Port : ActionPort  ActionPortLabel=case [ 75 76 77 78 79 80 81 82 83 84 85 86 87 88 89 90 91 92 93 94 95 96 97 98 99 100 ]:
  Out1 : Outport
  wires:
  In1/1 -> Out1/1

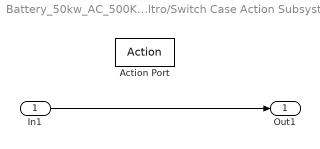
== system Battery_50kw_AC_500KW_400V_pruebas_2020_2_individual/Filtro/Switch Case Action Subsystem1 ==
  In1 : Inport
  Action Port : ActionPort  ActionPortLabel=case [ 45 46 47 48 49 50 51 52 53 54 55 56 57 58 59 60 61 62 63 64 65 66 67 68 69 70 ]:
  Out1 : Outport
  wires:
  In1/1 -> Out1/1

== system Battery_50kw_AC_500KW_400V_pruebas_2020_2_individual/Filtro/Switch Case Action Subsystem2 ==
  In1 : Inport
  Action Port : ActionPort  ActionPortLabel=default:
  Out1 : Outport
  wires:
  In1/1 -> Out1/1

== matlab function Battery_50kw_AC_500KW_400V_pruebas_2020_2_individual/MATLAB Function ==
  data: IN input; Current output; Enable output
%BLOQUE YA HECHO CON EL REPARTO 28/09/2023

function [Current,Enable]    = Ctr_V(IN)

 persistent val;
 
 if isempty(val)
     val=0;
 end
  
if IN >= 600
    Current =80;
    Enable= true;
    val=1;
elseif IN < 600 && val==1
    Current =80;
    Enable= true;
else
   Current=0;
   Enable=false;
end
    
 
% 
% function [Current,Enable]    = P_REG(IN)
% 
% persistent dato;
% 
% if isempty(dato)
%     dato=0;
%     
% end
%         
% if IN >= 550
%    dato=dato+10;
%    if dato>=50
%      Current = 80;
%      Enable=true;
%    else
%       Current=0;
%       Enable=false;
%    end      
% else
%    Current=0;
%    Enable=false;
% end
%

== matlab function Battery_50kw_AC_500KW_400V_pruebas_2020_2_individual/Filtro/MATLAB Function ==
  settings: updateMethod=DISCRETE
  data: Iabc input; inductancia output
%BLOQUE YA HECHO CON EL REPARTO 28/09/2023

function inductancia     = Ctr_Filtro(Iabc)

 persistent val;
 
 if isempty(val)
     val=0;
 end
  
if Iabc >= 70
    inductancia =5e-3;
    val=1;
   
else Iabc >= 30 && Iabc < 70 && val==1
    inductancia =8e-3;
    
%else
 %   inductancia=8e-3;
   %%inductancia=24e-3;%inductancia para 10kw
   %val=1;
end
    
 
% 
% function [Current,Enable]    = P_REG(IN)
% 
% persistent dato;
% 
% if isempty(dato)
%     dato=0;
%     
% end
%         
% if IN >= 550
%    dato=dato+10;
%    if dato>=50
%      Current = 80;
%      Enable=true;
%    else
%       Current=0;
%       Enable=false;
%    end      
% else
%    Current=0;
%    Enable=false;
% end
%
